simulink subsystem "VehicleEOMRef"  (R2024a)
settings: Solver=VariableStepAuto  StartTime=0.0  StopTime=10.0  RelTol=1e-3
undefined symbols (not defined in the file): Accel_bIi, AngularMomentum, AngularMomentumDot, Asensed_bIb, Forces, Moments, Omeg_BIb, Omeg_BIb_IC, OmegDtI_BIb, Pos_bii, Pos_bii_IC, Q_i2b, Q_i2b_IC, SimIn, SimPar, StateStruct, Vel_bEb_IC, Vel_bIi
libraries: starslibMathOperations x38, starslibAxisTransformations x25, starslibAirData x8, starslibKinematicalEquations x5, starslibGeodesy x4
(part 2 of 2)

== system VehicleEOMRef/Equations of Motion/Simple/State Labels ==
  I : Inport
  Bus Creator : BusCreator  Inputs=4
  Demux : Demux  Outputs=[3 3 3 4]
      settings: DisplayOption=none
  Reshape{1..3,5} (4 alike) : Reshape  OutputDimensionality=Column vector (2-D)
  O : Outport  VectorParamsAs1DForOutWhenUnconnected=off
  wires:
  Reshape5/1 -> Bus Creator/4  "Q_i2b"
  Reshape3/1 -> Bus Creator/3  "Pos_bii"
  Reshape2/1 -> Bus Creator/2  "Omeg_BIb"
  Reshape1/1 -> Bus Creator/1  "Vel_bEb"
  Demux/4 -> Reshape5/1  "Q_i2b"
  Demux/3 -> Reshape3/1  "Pos_bii"
  Demux/2 -> Reshape2/1  "Omeg_BIb"
  Demux/1 -> Reshape1/1  "Vel_bEb"
  Bus Creator/1 -> O/1
  I/1 -> Demux/1

== system VehicleEOMRef/Equations of Motion/Simple/Xdot Labels ==
  I : Inport
  Bus Creator : BusCreator  Inputs=4
  Demux : Demux  Outputs=[3 3 3 4]
      settings: DisplayOption=none
  O : Outport  VectorParamsAs1DForOutWhenUnconnected=off
  wires:
  Demux/4 -> Bus Creator/4  "QDt_i2b"
  Demux/3 -> Bus Creator/3  "PosDtI_bii"
  Demux/2 -> Bus Creator/2  "OmgDtI_BIb"
  Demux/1 -> Bus Creator/1  "VelDtB_bEb"
  I/1 -> Demux/1
  Bus Creator/1 -> O/1

== system VehicleEOMRef/Equations of Motion/STARS/Create STARS Inertial Reactions/RenameInertialReactionsBus ==
  Bus Creator2 : BusCreator  Inputs=4
  Constant{2..5} (4 alike) : Constant  Value=zeros(3,1)
  IR : Outport
  wires:
  Bus Creator2/1 -> IR/1  "InertialReactions"
  Constant5/1 -> Bus Creator2/4  "AngularMomentumDot"
  Constant2/1 -> Bus Creator2/1  "Forces"
  Constant4/1 -> Bus Creator2/3  "AngularMomentum"
  Constant3/1 -> Bus Creator2/2  "Moments"

== system VehicleEOMRef/Equations of Motion/STARS/Create STARS Initial Conditions/RenameIcOutputBus ==
  Bus Creator1 : BusCreator  Inputs=4
  Constant : Constant  Value=zeros(3,1)
  Constant1 : Constant  Value=zeros(3,1)
  Constant2 : Constant  Value=zeros(4,1)
  Constant4 : Constant  Value=zeros(3,1)
  Reshape{,1..3} (4 alike) : Reshape
  Out1 : Outport
  wires:
  Reshape1/1 -> Bus Creator1/2  "Vel_bEb_IC"
  Reshape2/1 -> Bus Creator1/3  "Q_i2b_IC"
  Reshape3/1 -> Bus Creator1/4  "Omeg_BIb_IC"
  Reshape/1 -> Bus Creator1/1  "Pos_bii_IC"
  Constant/1 -> Reshape/1
  Constant2/1 -> Reshape2/1
  Bus Creator1/1 -> Out1/1
  Constant1/1 -> Reshape1/1
  Constant4/1 -> Reshape3/1

== system VehicleEOMRef/Equations of Motion/STARS/Rigid Body Dynamics/Location ==
  note: Stevens & Lewis
      | 2nd ed.
      | eq. 1.5-16c
      | (NOT)
  note: Location
  Vel_bIi : Inport  PortDimensions=[3,1]
  Pos_bii_IC : Inport  Port=2  PortDimensions=[3,1]
  Reset : Inport  Port=3
  Inertial Position : Integrator  ExternalReset=either  InitialConditionSource=external  InitialCondition=StateStruct.PECI_ic_ft  ContinuousStateAttributes='Pos_bii'
  Pos_bii : Outport  PortDimensions=[3,1]
  wires:
  Vel_bIi/1 -> Inertial Position/1
  Inertial Position/1 -> Pos_bii/1  "Pos_bii"
  Reset/1 -> Inertial Position/2
  Pos_bii_IC/1 -> Inertial Position/3

== system VehicleEOMRef/Equations of Motion/STARS/Rigid Body Dynamics/Orientation ==
  note: Stevens & Lewis
      | 2nd ed.
      | eq. 1.5-16b
  note: Stevens & Lewis
      | 2nd ed.
      | eq. 1.5-16a
  note: Orientation
  Omega : Inport  PortDimensions=[3,1]
  Q_i2b_IC : Inport  Port=2  PortDimensions=[4,1]
  Reset : Inport  Port=3
  Inertial to Body Attitude : Integrator  ExternalReset=either  InitialConditionSource=external  InitialCondition=Q_i2b_IC  ContinuousStateAttributes='Q_i2b'
  Orthonormality Error : starslibMathOperations/Quaternion Propagation/Orthonormality Error  SystemSampleTime=-1  VariantActivationTime=update diagram  Latency=0  AutoFrameSizeCalculation=off
  Product : Product  RndMeth=Zero
  Quaternion Rate : starslibMathOperations/Quaternion Rate
  Sum : Sum  Inputs=|++
  k : Gain  Gain=K_QuatStab
  Q_i2b : Outport  PortDimensions=[4,1]
  wires:
  Omega/1 -> Quaternion Rate/2
  Quaternion Rate/1 -> Sum/1
  Orthonormality Error/1 -> k/1
  k/1 -> Product/1
  Product/1 -> Sum/2
  Inertial to Body Attitude/1 -> Product/2, Quaternion Rate/1, Orthonormality Error/1, Q_i2b/1  "Q_i2b"
  Reset/1 -> Inertial to Body Attitude/2
  Q_i2b_IC/1 -> Inertial to Body Attitude/3
  Sum/1 -> Inertial to Body Attitude/1

== system VehicleEOMRef/Equations of Motion/STARS/Rigid Body Dynamics/Rotation Rates ==
  note: Note:  This is the term for inertiaDot.  This may
      | not be valid for all cases where the inertia is
      | varying due to expelled mass (e.g. rocket
      | propellant).  It IS valid, however, in all cases where
      | the inertia is varying due to a geometric change
      | (e.g. deploying or inflatring a structure).
  note: Stevens & Lewis
      | 2nd ed.
      | eq. 1.5-16e
  note: Rotation Rates
  note: angular
      | momentum
  M : Inport  PortDimensions=[3,1]
  H : Inport  Port=2  PortDimensions=[3,1]
  Hdt : Inport  Port=3  PortDimensions=[3,1]
  I : Inport  Port=4  PortDimensions=[3,3]
  Iinv : Inport  Port=5  PortDimensions=[3,3]
  Idot : Inport  Port=6  PortDimensions=[3,3]
  Omeg_BIb_IC : Inport  Port=7
  Reset : Inport  Port=8
  Add : Sum
  Body Angular Rate : Integrator  ExternalReset=either  InitialConditionSource=external  InitialCondition=SimIn.EOM.Omeg_BIb  ContinuousStateAttributes='Omeg_BIb'
  Cross Product : starslibMathOperations/Cross Product
  IC switch : Constant  Value=IC_Accels
  Idotw : Product  Multiplication=Matrix(*)  SaturateOnIntegerOverflow=on  OutDataTypeStr=Inherit: Same as first input
  Iw : Product  Multiplication=Matrix(*)  SaturateOnIntegerOverflow=on  OutDataTypeStr=Inherit: Same as first input
  K_Idot : Gain  Gain=K_Idot
  Minv_times_vec : Product  Multiplication=Matrix(*)  SaturateOnIntegerOverflow=on  OutDataTypeStr=Inherit: Same as first input
  OmegaDot IC : InitialCondition  Value=OmegaDot_IC
  Switch : Switch  Criteria=u2 ~= 0  ZeroCross=off  SaturateOnIntegerOverflow=off  InputSameDT=off
  dif : Sum  Inputs=+---  InputSameDT=on  SaturateOnIntegerOverflow=on  OutDataTypeStr=Inherit: Same as first input
  OmegDtI_BIb : Outport  PortDimensions=[3,1]
  Omeg_BIb : Outport  Port=2  PortDimensions=[3,1]
  wires:
  Hdt/1 -> dif/4
  Switch/1 -> OmegDtI_BIb/1  "OmegDtI_BIb"
  Minv_times_vec/1 -> Body Angular Rate/1, Switch/3, OmegaDot IC/1  "OmegaDt_rps2"
  H/1 -> Add/2
  Add/1 -> Cross Product/2
  Cross Product/1 -> dif/2  "w_x_Iw"
  dif/1 -> Minv_times_vec/2
  M/1 -> dif/1
  Iw/1 -> Add/1
  I/1 -> Iw/1
  Iinv/1 -> Minv_times_vec/1
  Idot/1 -> Idotw/1
  Idotw/1 -> K_Idot/1
  Reset/1 -> Body Angular Rate/2
  Omeg_BIb_IC/1 -> Body Angular Rate/3
  Body Angular Rate/1 -> Iw/2, Cross Product/1, Idotw/2, Omeg_BIb/1  "Omeg_BIb"
  IC switch/1 -> Switch/2
  OmegaDot IC/1 -> Switch/1
  K_Idot/1 -> dif/3

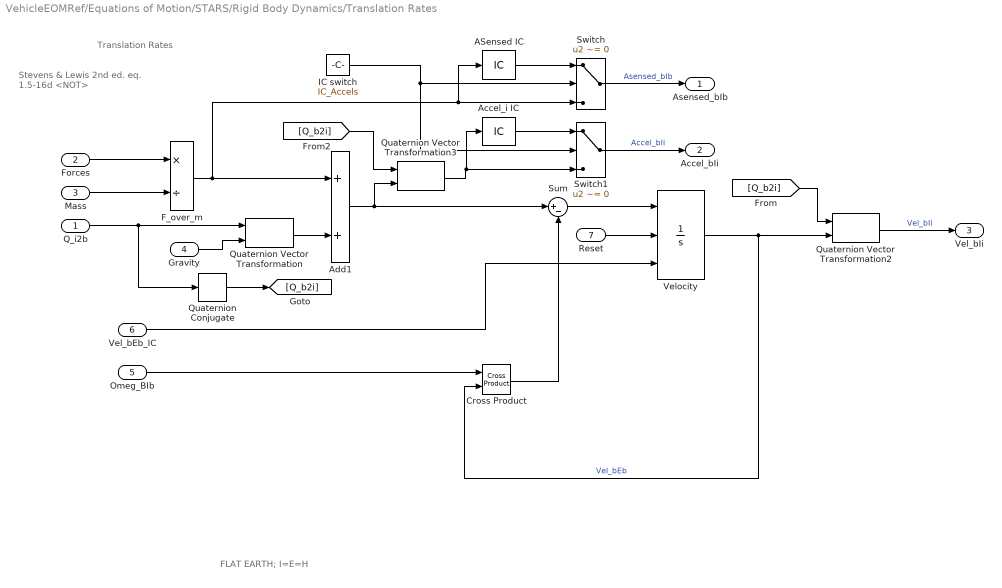
== system VehicleEOMRef/Equations of Motion/STARS/Rigid Body Dynamics/Translation Rates ==
  note: Stevens & Lewis
      | 2nd ed.
      | eq. 1.5-16d
      | <NOT>
  note: Translation Rates
  note: FLAT EARTH; I=E=H
  Q_i2b : Inport  PortDimensions=[4,1]
  Forces : Inport  Port=2  PortDimensions=[3,1]
  Mass : Inport  Port=3
  Gravity : Inport  Port=4
  Omeg_BIb : Inport  Port=5  PortDimensions=[3,1]
  Vel_bEb_IC : Inport  Port=6  PortDimensions=[3,1]
  Reset : Inport  Port=7
  ASensed IC : InitialCondition  Value=ASensed_IC
  Accel_i IC : InitialCondition  Value=Accel_i_IC
  Add1 : Sum
  Cross Product : starslibMathOperations/Cross Product
  F_over_m : Product  Inputs=*/  SaturateOnIntegerOverflow=on  OutDataTypeStr=Inherit: Same as first input
  IC switch : Constant  Value=IC_Accels
  Quaternion Conjugate : starslibMathOperations/Quaternion Conjugate  n=0
  Quaternion Vector Transformation : starslibAxisTransformations/Quaternion Vector Transformation  n=0
  Quaternion Vector Transformation2 : starslibAxisTransformations/Quaternion Vector Transformation  n=0
  Quaternion Vector Transformation3 : starslibAxisTransformations/Quaternion Vector Transformation  n=0
  Sum : Sum  Inputs=|+-
  Switch : Switch  Criteria=u2 ~= 0  ZeroCross=off  SaturateOnIntegerOverflow=off  InputSameDT=off
  Switch1 : Switch  Criteria=u2 ~= 0  ZeroCross=off  SaturateOnIntegerOverflow=off  InputSameDT=off
  Velocity : Integrator  ExternalReset=either  InitialConditionSource=external  InitialCondition=StateStruct.PECI_ic_ft  ContinuousStateAttributes='Vel_bEb'
  Asensed_bIb : Outport  PortDimensions=[3,1]
  Accel_bIi : Outport  Port=2  PortDimensions=[3,1]
  Vel_bIi : Outport  Port=3  PortDimensions=[3,1]
  wires:
  Quaternion Vector Transformation3/1 -> Switch1/3, Accel_i IC/1
  [Q_b2i] -> Quaternion Vector Transformation3/1
  Add1/1 -> Sum/1, Quaternion Vector Transformation3/2
  Quaternion Conjugate/1 -> [Q_b2i]
  Quaternion Vector Transformation/1 -> Add1/2
  Q_i2b/1 -> Quaternion Vector Transformation/1, Quaternion Conjugate/1
  Gravity/1 -> Quaternion Vector Transformation/2
  [Q_b2i] -> Quaternion Vector Transformation2/1
  Quaternion Vector Transformation2/1 -> Vel_bIi/1  "Vel_bIi"
  Sum/1 -> Velocity/1
  Cross Product/1 -> Sum/2
  Velocity/1 -> Cross Product/2, Quaternion Vector Transformation2/2  "Vel_bEb"
  Vel_bEb_IC/1 -> Velocity/3
  Omeg_BIb/1 -> Cross Product/1
  Switch/1 -> Asensed_bIb/1  "Asensed_bIb"
  Switch1/1 -> Accel_bIi/1  "Accel_bIi"
  F_over_m/1 -> Add1/1, Switch/3, ASensed IC/1
  Forces/1 -> F_over_m/1
  Mass/1 -> F_over_m/2
  Reset/1 -> Velocity/2
  ASensed IC/1 -> Switch/1
  Accel_i IC/1 -> Switch1/1
  IC switch/1 -> Switch1/2, Switch/2

== system VehicleEOMRef/Equations of Motion/Simple/Aircraft 6DOF/Quaternion Stabilization ==
  QuatDt : Inport  PortDimensions=[4,1]
  Quat_i2b : Inport  Port=2  PortDimensions=[4,1]
  Product : Product  InputSameDT=on  SaturateOnIntegerOverflow=on  OutDataTypeStr=Inherit: Same as first input
  Stab_gain : Subsystem
  Sum1 : Sum  Inputs=-+  InputSameDT=on  SaturateOnIntegerOverflow=on  OutDataTypeStr=Inherit: Same as first input
  qdot out : Outport  PortDimensions=[4,1]  VectorParamsAs1DForOutWhenUnconnected=off
  wires:
  Product/1 -> Sum1/1
  Stab_gain/1(stabilization_gain) -> Product/1
  Quat_i2b/1 -> Stab_gain/1(Quat_i2b), Product/2
  Sum1/1 -> qdot out/1
  QuatDt/1 -> Sum1/2

== system VehicleEOMRef/Equations of Motion/Simple/Aircraft 6DOF/quatDt ==
  pb_qb_rb : Inport  PortDimensions=[3,1]
  e0_eX_eY_eZ : Inport  Port=2  PortDimensions=[4,1]
  Gain : Gain  Gain=0.5  SaturateOnIntegerOverflow=on  OutDataTypeStr=Inherit: Same as input  ParamDataTypeStr=Inherit: Same as input
  Mux1 : Mux  Inputs=[3 4]
  Vector Concatenate : Concatenate  NumInputs=4  Mode=Multidimensional array
  e0dt : Fcn  Expr=-u[5]*u[1] - u[6]*u[2] - u[7]*u[3]
  eXdt : Fcn  Expr=u[4]*u[1] - u[7]*u[2] + u[6]*u[3]
  eYdt : Fcn  Expr=u[7]*u[1] + u[4]*u[2] - u[5]*u[3]
  eZdt : Fcn  Expr=-u[6]*u[1] + u[5]*u[2] + u[4]*u[3]
  e0D_eXD_eYD_eZD : Outport  PortDimensions=[4,1]  VectorParamsAs1DForOutWhenUnconnected=off
  wires:
  e0_eX_eY_eZ/1 -> Gain/1
  Vector Concatenate/1 -> e0D_eXD_eYD_eZD/1  "QuatDt_ps"
  e0dt/1 -> Vector Concatenate/1  "e0dt"
  eXdt/1 -> Vector Concatenate/2  "eXdt"
  eYdt/1 -> Vector Concatenate/3  "eYdt"
  Gain/1 -> Mux1/2
  pb_qb_rb/1 -> Mux1/1
  eZdt/1 -> Vector Concatenate/4  "eZdt"
  Mux1/1 -> eXdt/1, e0dt/1, eYdt/1, eZdt/1

== system VehicleEOMRef/Equations of Motion/Simple/Create Inertial Bus/RenameInertialBus ==
  Bus Creator : BusCreator  Inputs=7  OutDataTypeStr=Bus: InertialBus
  Constant{,1..5} (6 alike) : Constant  Value=zeros(3,1)  VectorParams1D=off
  Constant6 : Constant  Value=zeros(4,1)  VectorParams1D=off
  O : Outport  VectorParamsAs1DForOutWhenUnconnected=off
  wires:
  Constant6/1 -> Bus Creator/5  "Q_i2b"
  Constant2/1 -> Bus Creator/6  "Omeg_BIb"
  Constant5/1 -> Bus Creator/7  "OmegDtI_BIb"
  Bus Creator/1 -> O/1
  Constant4/1 -> Bus Creator/1  "Pos_bii"
  Constant/1 -> Bus Creator/2  "Vel_bIi"
  Constant1/1 -> Bus Creator/3  "Accel_bIi"
  Constant3/1 -> Bus Creator/4  "Asensed_bIb"

== system VehicleEOMRef/Equations of Motion/Simple/Aircraft 6DOF/Quaternion Stabilization/Stab_gain ==
  Quat_i2b : Inport  PortDimensions=[4,1]
  Constant : Constant  Value=1.0
  Demux : Demux
      settings: DisplayOption=none
  Gain1 : Gain  Gain=0.1  SaturateOnIntegerOverflow=on  OutDataTypeStr=Inherit: Same as input  ParamDataTypeStr=Inherit: Same as input
  Math Function{,1..3} (4 alike) : Math  Operator=square  SignedPower=on
  Sum1 : Sum  Inputs=4  SaturateOnIntegerOverflow=on
  Sum2 : Sum  Inputs=+-  SaturateOnIntegerOverflow=on
  stabilization_gain : Outport  PortDimensions=1  VectorParamsAs1DForOutWhenUnconnected=off
  wires:
  Quat_i2b/1 -> Demux/1
  Demux/4 -> Math Function3/1
  Demux/3 -> Math Function2/1
  Demux/2 -> Math Function1/1
  Demux/1 -> Math Function/1
  Gain1/1 -> stabilization_gain/1
  Sum2/1 -> Gain1/1
  Constant/1 -> Sum2/2
  Math Function3/1 -> Sum1/4
  Math Function2/1 -> Sum1/3
  Math Function1/1 -> Sum1/2
  Math Function/1 -> Sum1/1
  Sum1/1 -> Sum2/1
